simulink model "uavCtrltest0"  (Simulink 8.7)
settings: Solver=VariableStepAuto  StartTime=0.0  StopTime=1000  RelTol=1e-3
values from neighbouring files (symbols this model uses):
  utrim = [1.49457502486 3.95000888139e-15 -4.35170409107e-15 53.9352950493]    [data.mat]
settings Model: Creator=Administrator  LastModifiedBy=HFY12
settings DataIOCC: SignalLoggingSaveFormat=ModelDataLogs
settings OptimizationCC: ExpressionDepthLimit=2147483647  InitFltsAndDblsToZero=on
settings DebuggingCC: SolverPrmCheckMsg=warning  FcnCallInpInsideContextMsg=UseLocalSettings  StateNameClashWarn=warning
settings GRTTargetCC: GeneratePreprocessorConditionals=Use local settings  CombineOutputUpdateFcns=off  GRTInterface=on

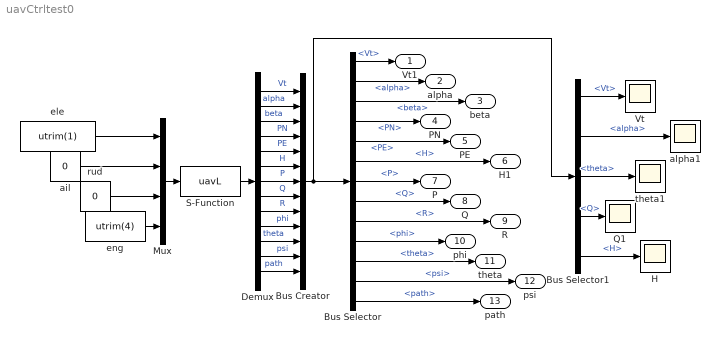
== system uavCtrltest0 ==
  Bus Creator : BusCreator  Inputs=13
  Bus Selector : BusSelector  OutputSignals=Vt,alpha,beta,PN,PE,H,P,Q,R,phi,theta,psi,path
  Bus Selector1 : BusSelector  OutputSignals=Vt,alpha,theta,Q,H
  Demux : Demux  Outputs=13
  H : Scope
  Mux : Mux
  Q1 : Scope
  S-Function : S-Function  FunctionName=uavL  SFunctionDeploymentMode=off  EnableBusSupport=off
  Vt : Scope
  ail : Constant  Value=0
  alpha1 : Scope
  ele : Constant  Value=utrim(1)
  eng : Constant  Value=utrim(4)
  rud : Constant  Value=0
  theta1 : Scope
  Vt1 : Outport
  alpha : Outport  Port=2
  beta : Outport  Port=3
  PN : Outport  Port=4
  PE : Outport  Port=5
  H1 : Outport  Port=6
  P : Outport  Port=7
  Q : Outport  Port=8
  R : Outport  Port=9
  phi : Outport  Port=10
  theta : Outport  Port=11
  psi : Outport  Port=12
  path : Outport  Port=13
  wires:
  Mux/1 -> S-Function/1
  ele/1 -> Mux/1
  ail/1 -> Mux/2
  rud/1 -> Mux/3
  eng/1 -> Mux/4
  S-Function/1 -> Demux/1
  Demux/1 -> Bus Creator/1  "Vt"
  Demux/2 -> Bus Creator/2  "alpha"
  Demux/3 -> Bus Creator/3  "beta"
  Demux/4 -> Bus Creator/4  "PN"
  Demux/5 -> Bus Creator/5  "PE"
  Demux/6 -> Bus Creator/6  "H"
  Demux/7 -> Bus Creator/7  "P"
  Demux/8 -> Bus Creator/8  "Q"
  Demux/9 -> Bus Creator/9  "R"
  Demux/10 -> Bus Creator/10  "phi"
  Demux/11 -> Bus Creator/11  "theta"
  Demux/12 -> Bus Creator/12  "psi"
  Demux/13 -> Bus Creator/13  "path"
  Bus Selector1/1 -> Vt/1  "<Vt>"
  Bus Selector1/2 -> alpha1/1  "<alpha>"
  Bus Selector1/3 -> theta1/1  "<theta>"
  Bus Selector1/4 -> Q1/1  "<Q>"
  Bus Selector1/5 -> H/1  "<H>"
  Bus Creator/1 -> Bus Selector/1, Bus Selector1/1
  Bus Selector/1 -> Vt1/1  "<Vt>"
  Bus Selector/2 -> alpha/1  "<alpha>"
  Bus Selector/3 -> beta/1  "<beta>"
  Bus Selector/4 -> PN/1  "<PN>"
  Bus Selector/13 -> path/1  "<path>"
  Bus Selector/12 -> psi/1  "<psi>"
  Bus Selector/11 -> theta/1  "<theta>"
  Bus Selector/10 -> phi/1  "<phi>"
  Bus Selector/9 -> R/1  "<R>"
  Bus Selector/8 -> Q/1  "<Q>"
  Bus Selector/7 -> P/1  "<P>"
  Bus Selector/6 -> H1/1  "<H>"
  Bus Selector/5 -> PE/1  "<PE>"
